simulink model "dio_eml"  (R2014a)
settings: Solver=FixedStepDiscrete  SolverMode=SingleTasking  StartTime=0.0  StopTime=10.0  RelTol=1e-3
settings Model: ExtModeTrigDuration=2  Creator=gcampa  LastModifiedBy=gcampa
settings OptimizationCC: OptimizeModelRefInitCode=on  LifeSpan=1  SimCompilerOptimization=off
settings DebuggingCC: UnderspecifiedInitializationDetection=Classic  SolverPrmCheckMsg=none  FrameProcessingCompatibilityMsg=error  StateNameClashWarn=warning
settings HardwareCC: ProdBitPerInt=16  ProdBitPerPointer=8  ProdIntDivRoundTo=Zero  ProdEndianess=LittleEndian  ProdWordSize=8  ProdHWDeviceType=Atmel->AVR
settings RTWCC: SystemTargetFile=realtime.tlc  GenerateMakefile=off  TemplateMakefile=realtime.tmf  Description=Run on Target Hardware  RTWVerbose=off  CustomSource=..\src\digitalio_arduino.cpp  RTWCompilerOptimization=off
settings STFCustomTargetCC: TargetLibSuffix=.a  GenerateSampleERTMain=on  ConcurrentExecutionCompliant=off  GeneratePreprocessorConditionals=Use local settings  ERTCustomFileBanners=on  SupportNonInlinedSFcns=off  SupportVariableSizeSignals=on  MATLABClassNameForMDSCustomization=Simulink.SoftwareTarget.ERTCustomization  GRTInterface=off  SystemTargetFile=realtime.tlc
settings ERTTargetCC: CombineOutputUpdateFcns=off  SupportContinuousTime=on  SupportVariableSizeSignals=on  ExtModeTransport=3  ExtModeMexFile=ext_serial_win32_comm  ExtModeMexArgs=0 1 9600  ERTSrcFileBannerTemplate=realtime_code_template.cgt  ERTHdrFileBannerTemplate=realtime_code_template.cgt  ERTDataSrcFileTemplate=realtime_code_template.cgt  ERTDataHdrFileTemplate=realtime_code_template.cgt  ERTCustomFileTemplate=realtime_file_process.tlc

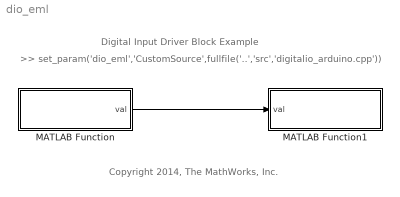
== system dio_eml ==
  note: Digital Input Driver Block Example
  note: Copyright 2014, The MathWorks, Inc.
  note: >> set_param('dio_eml','CustomSource',fullfile('..','src','digitalio_arduino.cpp'))
  MATLAB Function : MATLAB Function  TreatAsAtomicUnit=on  mask(Digital Read){pin=2, T=0.05}
      mask prompts: T "Sample Time"
      mask help:
      | Every time this block is executed it reads the digital value (0 or 1) of a given pin and sets it as the output of the block.
      |
      | The first parameter is the number of the pin where the digital input needs to be performed. The second parameter is the sample time.
      |
      | Note that if this block gets copied to a new model, then the file "digitalio_arduino.cpp" must be added to the CustomSource field of the new model using the "set_param" instruction. See the guide for more info.
  MATLAB Function1 : MATLAB Function  TreatAsAtomicUnit=on  mask(Digital Write){pin=3, T=0.05}
      mask prompts: T "Sample Time"
      mask help:
      | Every time this block is executed it gets the value (0 or 1) at its input and writes it (as a digital output) to a given pin.
      |
      | The first parameter is the number of the pin where the digital output needs to be performed. The second parameter is the sample time.
      |
      | Note that if this block gets copied to a new model, then the file "digitalio_arduino.cpp" must be added to the CustomSource field of the new model using the "set_param" instruction. See the guide for more info.
  wires:
  MATLAB Function/1(val) -> MATLAB Function1/1(val)

== matlab function dio_eml/MATLAB Function1 ==
  settings: updateMethod=DISCRETE  sampleTime=T
  data: pin parameter; in input
function digitalWrite(pin,in)
%#codegen

persistent initflag;

if strcmp(coder.target, 'rtw'),
    
    if isempty(initflag),
        % Initialize step
        coder.ceval('digitalIOSetup',uint8(pin),true);
        initflag = 1;
    else
        % output Step
        coder.ceval('writeDigitalPin',uint8(pin),logical(in));
    end
    
end

== matlab function dio_eml/MATLAB Function ==
  settings: updateMethod=DISCRETE  sampleTime=T
  data: pin parameter; out output
function out=digitalRead(pin)
%#codegen

persistent initflag;
out=0;

if strcmp(coder.target, 'rtw'),
    
    if isempty(initflag),
        % Initialize step
        coder.ceval('digitalIOSetup',uint8(pin),false);
        initflag = 1;
    else
        % output Step
        out=coder.ceval('readDigitalPin',uint8(pin));
    end
    
end

== matlab function dio_eml/MATLAB Function1 ==
  settings: updateMethod=DISCRETE  sampleTime=T
  data: pin parameter; val input
function digitalWrite(pin,val)
%#codegen

persistent initflag;

if strcmp(coder.target, 'rtw'),
    
    if isempty(initflag),
        % Initialize step
        coder.ceval('digitalIOSetup',uint8(pin),true);
        initflag = 1;
    else
        % output Step
        coder.ceval('writeDigitalPin',uint8(pin),logical(val));
    end
    
end

== matlab function dio_eml/MATLAB Function ==
  settings: updateMethod=DISCRETE  sampleTime=T
  data: pin parameter; val output
function val=digitalRead(pin)
%#codegen

persistent initflag;
val=0;

if strcmp(coder.target, 'rtw'),
    
    if isempty(initflag),
        % Initialize step
        coder.ceval('digitalIOSetup',uint8(pin),false);
        initflag = 1;
    else
        % output Step
        val=coder.ceval('readDigitalPin',uint8(pin));
    end
    
end
